simulink model "TypeA_siso180515"  (R2017b)
settings: Solver=ode45  StartTime=0.0  StopTime=12.0  RelTol=1e-3  EnableMultiTasking=on
undefined symbols (not defined in the file): cMat_BF, cMat_IM, cMat_MN, cMat_TM, gain_actBFGAS, gain_actBFL, gain_actBFP, gain_actBFR, gain_actBFT, gain_actBFV, gain_actBFY, gain_actF0GAS, gain_actF1GAS, gain_actF2GAS, gain_actF3GAS, gain_actIML, gain_actIMP, gain_actIMR, gain_actIMT, gain_actIMV, gain_actIMY, gain_actIPL, gain_actIPT, gain_actIPY, gain_actMNL, gain_actMNP, gain_actMNR, gain_actMNT, gain_actMNV, gain_actMNY, gain_actTML, gain_actTMP, gain_actTMY, gainBFGAS, gainBFL, gainBFP, gainBFR, gainBFT, gainBFV, gainBFY, gainF0GAS, gainF1GAS, gainF2GAS, gainF3GAS, gainHieBFP, gainHieBFR, gainHieBFY, gainHieIML, gainHieIMP, gainHieIMY, gainHieIPL, gainHieIPY, gainHieMNL, gainHieMNP, gainHieMNY, gainIML, gainIMP, gainIMR, gainIMT, gainIMV ... (+24)
libraries: cstblocks x57
(part 2 of 2)

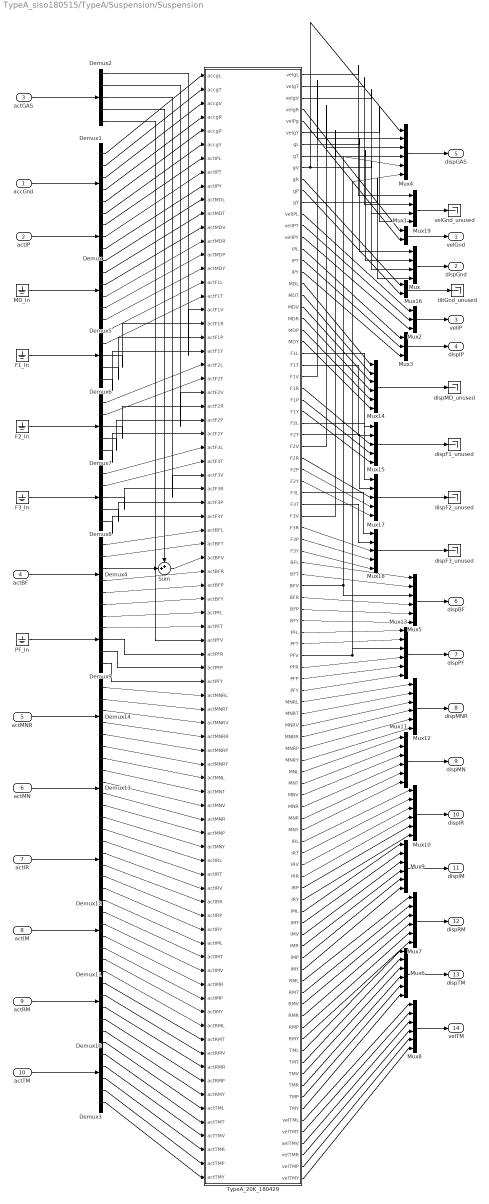
== system TypeA_siso180515/TypeA/Suspension/Suspension ==
  accGnd : Inport
  actIP : Inport  Port=2
  actGAS : Inport  Port=3
  actBF : Inport  Port=4
  actMNR : Inport  Port=5
  actMN : Inport  Port=6
  actIR : Inport  Port=7
  actIM : Inport  Port=8
  actRM : Inport  Port=9
  actTM : Inport  Port=10
  Demux : Demux  Outputs=3
  Demux{1,3..5,10..14} (9 alike) : Demux  Outputs=6
  Demux{2,6..9} (5 alike) : Demux  Outputs=5
  F1_In : Ground
  F2_In : Ground
  F3_In : Ground
  MD_In : Ground
  Mux : Mux
  Mux1 : Mux  Inputs=2
  Mux{4..14} (11 alike) : Mux  Inputs=6
  Mux15 : Mux  Inputs=5
  Mux16 : Mux  Inputs=2
  Mux17 : Mux  Inputs=5
  Mux18 : Mux  Inputs=5
  Mux19 : Mux
  Mux2 : Mux  Inputs=3
  Mux3 : Mux  Inputs=3
  PF_In : Ground
  Sum : Sum  Inputs=++|
  TypeA_20K_180429 : Subsystem
  dispF1_unused : Terminator
  dispF2_unused : Terminator
  dispF3_unused : Terminator
  dispMD_unused : Terminator
  tiltGnd_unused : Terminator
  velGnd_unused : Terminator
  velGnd : Outport
  dispGnd : Outport  Port=2
  velIP : Outport  Port=3
  dispIP : Outport  Port=4
  dispGAS : Outport  Port=5
  dispBF : Outport  Port=6
  dispPF : Outport  Port=7
  dispMNR : Outport  Port=8
  dispMN : Outport  Port=9
  dispIR : Outport  Port=10
  dispIM : Outport  Port=11
  dispRM : Outport  Port=12
  dispTM : Outport  Port=13
  velTM : Outport  Port=14
  wires:
  Mux/1 -> dispGnd/1
  Mux1/1 -> velGnd/1
  Mux2/1 -> velIP/1
  Mux3/1 -> dispIP/1
  Mux4/1 -> dispGAS/1
  Mux5/1 -> dispBF/1
  Mux6/1 -> dispTM/1
  actIP/1 -> Demux/1
  accGnd/1 -> Demux1/1
  actTM/1 -> Demux3/1
  Demux4/3 -> Sum/2
  Demux2/4 -> Sum/1
  Demux2/5 -> TypeA_20K_180429/42(actPFV)
  actBF/1 -> Demux4/1
  actGAS/1 -> Demux2/1
  Demux1/3 -> TypeA_20K_180429/3(accgV)
  Demux1/1 -> TypeA_20K_180429/1(accgL)
  Demux1/2 -> TypeA_20K_180429/2(accgT)
  Demux1/4 -> TypeA_20K_180429/4(accgR)
  Demux1/5 -> TypeA_20K_180429/5(accgP)
  Demux1/6 -> TypeA_20K_180429/6(accgY)
  Demux/1 -> TypeA_20K_180429/7(actIPL)
  Demux/2 -> TypeA_20K_180429/8(actIPT)
  Demux/3 -> TypeA_20K_180429/9(actIPY)
  MD_In/1 -> Demux5/1
  Demux5/1 -> TypeA_20K_180429/10(actMDL)
  Demux5/2 -> TypeA_20K_180429/11(actMDT)
  Demux5/3 -> TypeA_20K_180429/12(actMDV)
  Demux5/4 -> TypeA_20K_180429/13(actMDR)
  Demux5/5 -> TypeA_20K_180429/14(actMDP)
  Demux5/6 -> TypeA_20K_180429/15(actMDY)
  Demux2/1 -> TypeA_20K_180429/18(actF1V)
  Demux2/2 -> TypeA_20K_180429/24(actF2V)
  Demux2/3 -> TypeA_20K_180429/30(actF3V)
  Sum/1 -> TypeA_20K_180429/36(actBFV)
  F1_In/1 -> Demux6/1
  Demux6/2 -> TypeA_20K_180429/17(actF1T)
  Demux6/1 -> TypeA_20K_180429/16(actF1L)
  Demux6/5 -> TypeA_20K_180429/21(actF1Y)
  Demux6/3 -> TypeA_20K_180429/19(actF1R)
  Demux6/4 -> TypeA_20K_180429/20(actF1P)
  F2_In/1 -> Demux7/1
  Demux7/1 -> TypeA_20K_180429/22(actF2L)
  Demux7/2 -> TypeA_20K_180429/23(actF2T)
  Demux7/3 -> TypeA_20K_180429/25(actF2R)
  Demux7/4 -> TypeA_20K_180429/26(actF2P)
  Demux7/5 -> TypeA_20K_180429/27(actF2Y)
  F3_In/1 -> Demux8/1
  Demux8/2 -> TypeA_20K_180429/29(actF3T)
  Demux8/1 -> TypeA_20K_180429/28(actF3L)
  Demux8/5 -> TypeA_20K_180429/33(actF3Y)
  Demux8/4 -> TypeA_20K_180429/32(actF3P)
  Demux8/3 -> TypeA_20K_180429/31(actF3R)
  Demux4/1 -> TypeA_20K_180429/34(actBFL)
  Demux4/2 -> TypeA_20K_180429/35(actBFT)
  Demux4/4 -> TypeA_20K_180429/37(actBFR)
  Demux4/5 -> TypeA_20K_180429/38(actBFP)
  Demux4/6 -> TypeA_20K_180429/39(actBFY)
  PF_In/1 -> Demux9/1
  Demux9/1 -> TypeA_20K_180429/40(actPFL)
  Demux9/2 -> TypeA_20K_180429/41(actPFT)
  Demux9/4 -> TypeA_20K_180429/44(actPFP)
  Demux9/3 -> TypeA_20K_180429/43(actPFR)
  Demux9/5 -> TypeA_20K_180429/45(actPFY)
  actRM/1 -> Demux10/1
  actIM/1 -> Demux11/1
  actIR/1 -> Demux12/1
  actMN/1 -> Demux13/1
  actMNR/1 -> Demux14/1
  Demux14/4 -> TypeA_20K_180429/49(actMNRR)
  Demux14/5 -> TypeA_20K_180429/50(actMNRP)
  Demux14/6 -> TypeA_20K_180429/51(actMNRY)
  Demux14/1 -> TypeA_20K_180429/46(actMNRL)
  Demux14/2 -> TypeA_20K_180429/47(actMNRT)
  Demux14/3 -> TypeA_20K_180429/48(actMNRV)
  Demux13/2 -> TypeA_20K_180429/53(actMNT)
  Demux13/1 -> TypeA_20K_180429/52(actMNL)
  Demux13/3 -> TypeA_20K_180429/54(actMNV)
  Demux13/5 -> TypeA_20K_180429/56(actMNP)
  Demux13/4 -> TypeA_20K_180429/55(actMNR)
  Demux13/6 -> TypeA_20K_180429/57(actMNY)
  Demux12/6 -> TypeA_20K_180429/63(actIRY)
  Demux12/2 -> TypeA_20K_180429/59(actIRT)
  Demux12/5 -> TypeA_20K_180429/62(actIRP)
  Demux12/3 -> TypeA_20K_180429/60(actIRV)
  Demux12/4 -> TypeA_20K_180429/61(actIRR)
  Demux12/1 -> TypeA_20K_180429/58(actIRL)
  Demux11/2 -> TypeA_20K_180429/65(actIMT)
  Demux11/3 -> TypeA_20K_180429/66(actIMV)
  Demux11/5 -> TypeA_20K_180429/68(actIMP)
  Demux11/4 -> TypeA_20K_180429/67(actIMR)
  Demux11/1 -> TypeA_20K_180429/64(actIML)
  Demux11/6 -> TypeA_20K_180429/69(actIMY)
  Demux10/5 -> TypeA_20K_180429/74(actRMP)
  Demux10/6 -> TypeA_20K_180429/75(actRMY)
  Demux10/4 -> TypeA_20K_180429/73(actRMR)
  Demux10/3 -> TypeA_20K_180429/72(actRMV)
  Demux10/1 -> TypeA_20K_180429/70(actRML)
  Demux10/2 -> TypeA_20K_180429/71(actRMT)
  Demux3/3 -> TypeA_20K_180429/78(actTMV)
  Demux3/1 -> TypeA_20K_180429/76(actTML)
  Demux3/2 -> TypeA_20K_180429/77(actTMT)
  Demux3/4 -> TypeA_20K_180429/79(actTMR)
  Demux3/5 -> TypeA_20K_180429/80(actTMP)
  Demux3/6 -> TypeA_20K_180429/81(actTMY)
  Mux7/1 -> dispRM/1
  Mux8/1 -> velTM/1
  Mux9/1 -> dispIM/1
  Mux10/1 -> dispIR/1
  Mux11/1 -> dispMN/1
  Mux12/1 -> dispMNR/1
  Mux13/1 -> dispPF/1
  Mux14/1 -> dispMD_unused/1
  Mux15/1 -> dispF1_unused/1
  Mux16/1 -> tiltGnd_unused/1
  Mux17/1 -> dispF2_unused/1
  Mux18/1 -> dispF3_unused/1
  TypeA_20K_180429/4(velgR) -> Mux1/1
  TypeA_20K_180429/5(velPg) -> Mux1/2
  TypeA_20K_180429/8(gT) -> Mux/2
  TypeA_20K_180429/7(gL) -> Mux/1
  TypeA_20K_180429/9(gV) -> Mux/3, Mux4/1
  TypeA_20K_180429/11(gP) -> Mux16/2
  TypeA_20K_180429/10(gR) -> Mux16/1
  TypeA_20K_180429/12(gY) -> Mux/4
  TypeA_20K_180429/14(velIPT) -> Mux2/2
  TypeA_20K_180429/15(velIPY) -> Mux2/3
  TypeA_20K_180429/13(velIPL) -> Mux2/1
  TypeA_20K_180429/17(IPT) -> Mux3/2
  TypeA_20K_180429/16(IPL) -> Mux3/1
  TypeA_20K_180429/18(IPY) -> Mux3/3
  TypeA_20K_180429/19(MDL) -> Mux14/1
  TypeA_20K_180429/21(MDV) -> Mux14/3
  TypeA_20K_180429/20(MDT) -> Mux14/2
  TypeA_20K_180429/22(MDR) -> Mux14/4
  TypeA_20K_180429/23(MDP) -> Mux14/5
  TypeA_20K_180429/24(MDY) -> Mux14/6
  TypeA_20K_180429/27(F1V) -> Mux4/2
  TypeA_20K_180429/33(F2V) -> Mux4/3
  TypeA_20K_180429/39(F3V) -> Mux4/4
  TypeA_20K_180429/45(BFV) -> Mux4/5, Mux5/3
  TypeA_20K_180429/51(PFV) -> Mux4/6, Mux13/3
  TypeA_20K_180429/25(F1L) -> Mux15/1
  TypeA_20K_180429/26(F1T) -> Mux15/2
  TypeA_20K_180429/30(F1Y) -> Mux15/5
  TypeA_20K_180429/28(F1R) -> Mux15/3
  TypeA_20K_180429/29(F1P) -> Mux15/4
  TypeA_20K_180429/31(F2L) -> Mux17/1
  TypeA_20K_180429/32(F2T) -> Mux17/2
  TypeA_20K_180429/34(F2R) -> Mux17/3
  TypeA_20K_180429/36(F2Y) -> Mux17/5
  TypeA_20K_180429/35(F2P) -> Mux17/4
  TypeA_20K_180429/37(F3L) -> Mux18/1
  TypeA_20K_180429/38(F3T) -> Mux18/2
  TypeA_20K_180429/42(F3Y) -> Mux18/5
  TypeA_20K_180429/41(F3P) -> Mux18/4
  TypeA_20K_180429/40(F3R) -> Mux18/3
  TypeA_20K_180429/47(BFP) -> Mux5/5
  TypeA_20K_180429/48(BFY) -> Mux5/6
  TypeA_20K_180429/46(BFR) -> Mux5/4
  TypeA_20K_180429/44(BFT) -> Mux5/2
  TypeA_20K_180429/43(BFL) -> Mux5/1
  TypeA_20K_180429/54(PFY) -> Mux13/6
  TypeA_20K_180429/49(PFL) -> Mux13/1
  TypeA_20K_180429/50(PFT) -> Mux13/2
  TypeA_20K_180429/52(PFR) -> Mux13/4
  TypeA_20K_180429/53(PFP) -> Mux13/5
  TypeA_20K_180429/56(MNRT) -> Mux12/2
  TypeA_20K_180429/60(MNRY) -> Mux12/6
  TypeA_20K_180429/57(MNRV) -> Mux12/3
  TypeA_20K_180429/58(MNRR) -> Mux12/4
  TypeA_20K_180429/55(MNRL) -> Mux12/1
  TypeA_20K_180429/59(MNRP) -> Mux12/5
  TypeA_20K_180429/64(MNR) -> Mux11/4
  TypeA_20K_180429/61(MNL) -> Mux11/1
  TypeA_20K_180429/63(MNV) -> Mux11/3
  TypeA_20K_180429/62(MNT) -> Mux11/2
  TypeA_20K_180429/66(MNY) -> Mux11/6
  TypeA_20K_180429/65(MNP) -> Mux11/5
  TypeA_20K_180429/71(IRP) -> Mux10/5
  TypeA_20K_180429/69(IRV) -> Mux10/3
  TypeA_20K_180429/72(IRY) -> Mux10/6
  TypeA_20K_180429/70(IRR) -> Mux10/4
  TypeA_20K_180429/68(IRT) -> Mux10/2
  TypeA_20K_180429/67(IRL) -> Mux10/1
  TypeA_20K_180429/73(IML) -> Mux9/1
  TypeA_20K_180429/75(IMV) -> Mux9/3
  TypeA_20K_180429/74(IMT) -> Mux9/2
  TypeA_20K_180429/76(IMR) -> Mux9/4
  TypeA_20K_180429/77(IMP) -> Mux9/5
  TypeA_20K_180429/78(IMY) -> Mux9/6
  TypeA_20K_180429/83(RMP) -> Mux7/5
  TypeA_20K_180429/84(RMY) -> Mux7/6
  TypeA_20K_180429/79(RML) -> Mux7/1
  TypeA_20K_180429/81(RMV) -> Mux7/3
  TypeA_20K_180429/80(RMT) -> Mux7/2
  TypeA_20K_180429/82(RMR) -> Mux7/4
  TypeA_20K_180429/85(TML) -> Mux6/1
  TypeA_20K_180429/86(TMT) -> Mux6/2
  TypeA_20K_180429/88(TMR) -> Mux6/4
  TypeA_20K_180429/87(TMV) -> Mux6/3
  TypeA_20K_180429/89(TMP) -> Mux6/5
  TypeA_20K_180429/90(TMY) -> Mux6/6
  TypeA_20K_180429/93(velTMV) -> Mux8/3
  TypeA_20K_180429/94(velTMR) -> Mux8/4
  TypeA_20K_180429/96(velTMY) -> Mux8/6
  TypeA_20K_180429/91(velTML) -> Mux8/1
  TypeA_20K_180429/95(velTMP) -> Mux8/5
  TypeA_20K_180429/92(velTMT) -> Mux8/2
  Mux19/1 -> velGnd_unused/1
  TypeA_20K_180429/1(velgL) -> Mux19/1
  TypeA_20K_180429/2(velgT) -> Mux19/2
  TypeA_20K_180429/3(velgV) -> Mux19/3
  TypeA_20K_180429/6(velgY) -> Mux19/4

== system TypeA_siso180515/TypeA/Suspension/aMatrix_BF ==
  aMat_in : Inport
  cMat_BF : Constant  Value=cMat_BF  VectorParams1D=off
  coupling_BF : Product  Multiplication=Matrix(*)
  actBF : Outport
  wires:
  coupling_BF/1 -> actBF/1
  aMat_in/1 -> coupling_BF/2
  cMat_BF/1 -> coupling_BF/1

== system TypeA_siso180515/TypeA/Suspension/aMatrix_GAS ==
  aMat_in : Inport
  Add{1..4} (4 alike) : Sum  Inputs=+-
  Demux4 : Demux  Outputs=5
  Mux3 : Mux  Inputs=5
  actGAS : Outport
  wires:
  aMat_in/1 -> Demux4/1
  Mux3/1 -> actGAS/1
  Add1/1 -> Mux3/1
  Add2/1 -> Mux3/2
  Demux4/3 -> Add3/1, Add2/2
  Demux4/2 -> Add1/2, Add2/1
  Demux4/1 -> Add1/1
  Demux4/5 -> Mux3/5, Add4/2
  Add4/1 -> Mux3/4
  Add3/1 -> Mux3/3
  Demux4/4 -> Add3/2, Add4/1

== system TypeA_siso180515/TypeA/Suspension/aMatrix_IM ==
  aMat_in : Inport
  Gain : Gain  Gain=-1
  cMat_IM : Constant  Value=cMat_IM  VectorParams1D=off
  coupling_IM : Product  Multiplication=Matrix(*)
  actIR : Outport
  actIM : Outport  Port=2
  wires:
  coupling_IM/1 -> actIM/1, Gain/1
  aMat_in/1 -> coupling_IM/2
  cMat_IM/1 -> coupling_IM/1
  Gain/1 -> actIR/1

== system TypeA_siso180515/TypeA/Suspension/aMatrix_MN ==
  aMat_in : Inport
  Gain : Gain  Gain=-1
  cMat_MN : Constant  Value=cMat_MN  VectorParams1D=off
  coupling_MN : Product  Multiplication=Matrix(*)
  actMNR : Outport
  actMN : Outport  Port=2
  wires:
  coupling_MN/1 -> actMN/1, Gain/1
  aMat_in/1 -> coupling_MN/2
  cMat_MN/1 -> coupling_MN/1
  Gain/1 -> actMNR/1

== system TypeA_siso180515/TypeA/Suspension/aMatrix_TM ==
  aMat_in : Inport
  Demux : Demux  Outputs=3
  Demux1 : Demux  Outputs=3
  Gain : Gain  Gain=-1
  Ground{,1..5} (6 alike) : Ground
  Mux : Mux  Inputs=6
  Mux1 : Mux  Inputs=6
  cMat_TM : Constant  Value=cMat_TM  VectorParams1D=off
  coupling_TM : Product  Multiplication=Matrix(*)
  actRM : Outport
  actTM : Outport  Port=2
  wires:
  coupling_TM/1 -> Demux1/1, Gain/1
  aMat_in/1 -> coupling_TM/2  "3DoF"
  cMat_TM/1 -> coupling_TM/1
  Gain/1 -> Demux/1
  Demux/1 -> Mux/1
  Demux/2 -> Mux/5
  Demux/3 -> Mux/6
  Demux1/1 -> Mux1/1
  Demux1/3 -> Mux1/6
  Demux1/2 -> Mux1/5
  Ground/1 -> Mux/2
  Ground1/1 -> Mux/3
  Ground2/1 -> Mux/4
  Ground4/1 -> Mux1/3
  Ground3/1 -> Mux1/2
  Ground5/1 -> Mux1/4
  Mux/1 -> actRM/1  "6DoF"
  Mux1/1 -> actTM/1  "6DoF"

== system TypeA_siso180515/TypeA/Suspension/sMatrix_BF_LVDT ==
  dispGnd : Inport
  dispBF : Inport  Port=2
  Add2 : Sum  Inputs=-+
  Demux : Demux
  Ground : Ground
  Ground1 : Ground
  Mux : Mux  Inputs=6
  BF_LVDT : Outport
  wires:
  Add2/1 -> BF_LVDT/1  "6DoF"
  dispBF/1 -> Add2/2  "6DoF"
  dispGnd/1 -> Demux/1  "4DoF"
  Demux/1 -> Mux/1  "L"
  Demux/2 -> Mux/2  "T"
  Demux/3 -> Mux/3  "V"
  Demux/4 -> Mux/6  "Y"
  Ground/1 -> Mux/4  "R"
  Ground1/1 -> Mux/5  "P"
  Mux/1 -> Add2/1

== system TypeA_siso180515/TypeA/Suspension/sMatrix_GAS_LVDT ==
  dispGAS : Inport
  Add{1..5} (5 alike) : Sum  Inputs=-+
  Demux4 : Demux  Outputs=6
  Mux3 : Mux  Inputs=5
  GAS_LVDT : Outport
  wires:
  dispGAS/1 -> Demux4/1
  Demux4/1 -> Add2/1  "VGnd = IPV"
  Demux4/2 -> Add1/1, Add2/2  "VF1"
  Demux4/3 -> Add1/2, Add3/1  "VF2"
  Demux4/4 -> Add4/1, Add3/2  "VF3"
  Add2/1 -> Mux3/1  "GASF0"
  Add1/1 -> Mux3/2  "GASF1"
  Add3/1 -> Mux3/3  "GASF2"
  Mux3/1 -> GAS_LVDT/1
  Demux4/5 -> Add5/1, Add4/2  "VBF"
  Demux4/6 -> Add5/2  "VPF"
  Add4/1 -> Mux3/4  "GASF3"
  Add5/1 -> Mux3/5  "GASBF"

== system TypeA_siso180515/TypeA/Suspension/sMatrix_IM_PS ==
  dispIR : Inport
  dispIM : Inport  Port=2
  Add2 : Sum  Inputs=-+
  IM_PS : Outport
  wires:
  Add2/1 -> IM_PS/1
  dispIM/1 -> Add2/2
  dispIR/1 -> Add2/1

== system TypeA_siso180515/TypeA/Suspension/sMatrix_IP_LVDT ==
  dispGnd : Inport
  dispIP : Inport  Port=2
  Add2 : Sum  Inputs=-+
  Demux : Demux
  Mux : Mux  Inputs=3
  Terminator : Terminator
  IP_LVDT : Outport
  wires:
  Add2/1 -> IP_LVDT/1
  dispIP/1 -> Add2/2
  dispGnd/1 -> Demux/1
  Demux/1 -> Mux/1  "L"
  Demux/2 -> Mux/2  "T"
  Demux/4 -> Mux/3  "Y"
  Demux/3 -> Terminator/1  "V"
  Mux/1 -> Add2/1

== system TypeA_siso180515/TypeA/Suspension/sMatrix_MN_OpLev ==
  dispMN : Inport
  Demux4 : Demux  Outputs=6
  Mux3 : Mux  Inputs=3
  dispMNL : Terminator
  dispMNT : Terminator
  dispMNV : Terminator
  MN_OpLev : Outport
  wires:
  dispMN/1 -> Demux4/1
  Mux3/1 -> MN_OpLev/1
  Demux4/1 -> dispMNL/1
  Demux4/2 -> dispMNT/1
  Demux4/3 -> dispMNV/1
  Demux4/4 -> Mux3/1
  Demux4/5 -> Mux3/2
  Demux4/6 -> Mux3/3

== system TypeA_siso180515/TypeA/Suspension/sMatrix_MN_PS ==
  dispMNR : Inport
  dispMN : Inport  Port=2
  Add2 : Sum  Inputs=-+
  MN_PS : Outport
  wires:
  Add2/1 -> MN_PS/1
  dispMN/1 -> Add2/2
  dispMNR/1 -> Add2/1

== system TypeA_siso180515/TypeA/Suspension/sMatrix_PF_OpLev ==
  dispPF : Inport
  Demux4 : Demux  Outputs=6
  Mux3 : Mux  Inputs=3
  dispLPF : Terminator
  dispTPF : Terminator
  dispVPF : Terminator
  OpLev_PF : Outport
  wires:
  dispPF/1 -> Demux4/1
  Mux3/1 -> OpLev_PF/1
  Demux4/1 -> dispLPF/1
  Demux4/2 -> dispTPF/1
  Demux4/3 -> dispVPF/1
  Demux4/4 -> Mux3/1
  Demux4/5 -> Mux3/2
  Demux4/6 -> Mux3/3

== system TypeA_siso180515/TypeA/Suspension/sMatrix_TM_OpLev ==
  dispTM : Inport
  Demux4 : Demux  Outputs=6
  Mux3 : Mux  Inputs=3
  dispTMR : Terminator
  dispTMT : Terminator
  dispTMV : Terminator
  TM_OpLev : Outport
  wires:
  dispTM/1 -> Demux4/1
  Mux3/1 -> TM_OpLev/1
  Demux4/1 -> Mux3/1
  Demux4/2 -> dispTMT/1
  Demux4/3 -> dispTMV/1
  Demux4/4 -> dispTMR/1
  Demux4/5 -> Mux3/2
  Demux4/6 -> Mux3/3

== system TypeA_siso180515/TypeA/Suspension/sMatrix_TM_PS ==
  dispRM : Inport
  dispTM : Inport  Port=2
  Add2 : Sum  Inputs=-+
  Demux : Demux  Outputs=6
  Demux1 : Demux  Outputs=6
  Mux : Mux  Inputs=3
  Mux1 : Mux  Inputs=3
  Terminator{,1..5} (6 alike) : Terminator
  TM_PS : Outport
  wires:
  Add2/1 -> TM_PS/1  "(L, P, Y)"
  dispRM/1 -> Demux/1
  dispTM/1 -> Demux1/1
  Demux/1 -> Mux/1  "L"
  Demux/5 -> Mux/2  "P"
  Demux/6 -> Mux/3  "Y"
  Demux1/1 -> Mux1/1  "L"
  Demux1/5 -> Mux1/2  "P"
  Demux1/6 -> Mux1/3  "Y"
  Mux/1 -> Add2/1
  Mux1/1 -> Add2/2
  Demux/2 -> Terminator/1  "T"
  Demux/4 -> Terminator2/1  "R"
  Demux/3 -> Terminator1/1  "V"
  Demux1/4 -> Terminator5/1  "R"
  Demux1/2 -> Terminator3/1  "T"
  Demux1/3 -> Terminator4/1  "V"

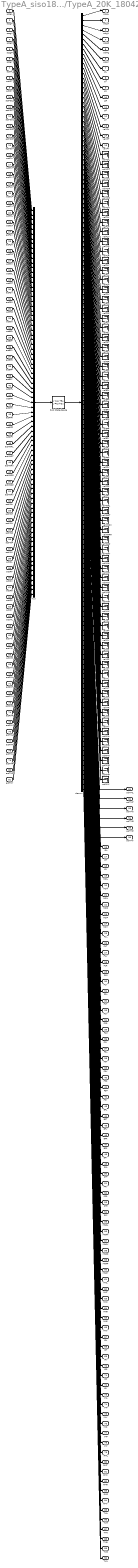
== system TypeA_siso180515/TypeA/Suspension/Suspension/TypeA_20K_180429 ==
  accgL : Inport
  accgT : Inport  Port=2
  accgV : Inport  Port=3
  accgR : Inport  Port=4
  accgP : Inport  Port=5
  accgY : Inport  Port=6
  actIPL : Inport  Port=7
  actIPT : Inport  Port=8
  actIPY : Inport  Port=9
  actMDL : Inport  Port=10
  actMDT : Inport  Port=11
  actMDV : Inport  Port=12
  actMDR : Inport  Port=13
  actMDP : Inport  Port=14
  actMDY : Inport  Port=15
  actF1L : Inport  Port=16
  actF1T : Inport  Port=17
  actF1V : Inport  Port=18
  actF1R : Inport  Port=19
  actF1P : Inport  Port=20
  actF1Y : Inport  Port=21
  actF2L : Inport  Port=22
  actF2T : Inport  Port=23
  actF2V : Inport  Port=24
  actF2R : Inport  Port=25
  actF2P : Inport  Port=26
  actF2Y : Inport  Port=27
  actF3L : Inport  Port=28
  actF3T : Inport  Port=29
  actF3V : Inport  Port=30
  actF3R : Inport  Port=31
  actF3P : Inport  Port=32
  actF3Y : Inport  Port=33
  actBFL : Inport  Port=34
  actBFT : Inport  Port=35
  actBFV : Inport  Port=36
  actBFR : Inport  Port=37
  actBFP : Inport  Port=38
  actBFY : Inport  Port=39
  actPFL : Inport  Port=40
  actPFT : Inport  Port=41
  actPFV : Inport  Port=42
  actPFR : Inport  Port=43
  actPFP : Inport  Port=44
  actPFY : Inport  Port=45
  actMNRL : Inport  Port=46
  actMNRT : Inport  Port=47
  actMNRV : Inport  Port=48
  actMNRR : Inport  Port=49
  actMNRP : Inport  Port=50
  actMNRY : Inport  Port=51
  actMNL : Inport  Port=52
  actMNT : Inport  Port=53
  actMNV : Inport  Port=54
  actMNR : Inport  Port=55
  actMNP : Inport  Port=56
  actMNY : Inport  Port=57
  actIRL : Inport  Port=58
  actIRT : Inport  Port=59
  actIRV : Inport  Port=60
  actIRR : Inport  Port=61
  actIRP : Inport  Port=62
  actIRY : Inport  Port=63
  actIML : Inport  Port=64
  actIMT : Inport  Port=65
  actIMV : Inport  Port=66
  actIMR : Inport  Port=67
  actIMP : Inport  Port=68
  actIMY : Inport  Port=69
  actRML : Inport  Port=70
  actRMT : Inport  Port=71
  actRMV : Inport  Port=72
  actRMR : Inport  Port=73
  actRMP : Inport  Port=74
  actRMY : Inport  Port=75
  actTML : Inport  Port=76
  actTMT : Inport  Port=77
  actTMV : Inport  Port=78
  actTMR : Inport  Port=79
  actTMP : Inport  Port=80
  actTMY : Inport  Port=81
  SAS State-Space : StateSpace  A=sys1.A  B=sys1.B  C=sys1.C  D=sys1.D  InitialCondition=0  ContinuousStateAttributes='SUS_SS_MODEL'
  demux : Demux  Outputs=162
  mux : Mux  Inputs=81
  velBFL : Terminator
  velBFP : Terminator
  velBFR : Terminator
  velBFT : Terminator
  velBFV : Terminator
  velBFY : Terminator
  velF1L : Terminator
  velF1P : Terminator
  velF1R : Terminator
  velF1T : Terminator
  velF1V : Terminator
  velF1Y : Terminator
  velF2L : Terminator
  velF2P : Terminator
  velF2R : Terminator
  velF2T : Terminator
  velF2V : Terminator
  velF2Y : Terminator
  velF3L : Terminator
  velF3P : Terminator
  velF3R : Terminator
  velF3T : Terminator
  velF3V : Terminator
  velF3Y : Terminator
  velIML : Terminator
  velIMP : Terminator
  velIMR : Terminator
  velIMT : Terminator
  velIMV : Terminator
  velIMY : Terminator
  velIRL : Terminator
  velIRP : Terminator
  velIRR : Terminator
  velIRT : Terminator
  velIRV : Terminator
  velIRY : Terminator
  velMDL : Terminator
  velMDP : Terminator
  velMDR : Terminator
  velMDT : Terminator
  velMDV : Terminator
  velMDY : Terminator
  velMNL : Terminator
  velMNP : Terminator
  velMNR : Terminator
  velMNRL : Terminator
  velMNRP : Terminator
  velMNRR : Terminator
  velMNRT : Terminator
  velMNRV : Terminator
  velMNRY : Terminator
  velMNT : Terminator
  velMNV : Terminator
  velMNY : Terminator
  velPFL : Terminator
  velPFP : Terminator
  velPFR : Terminator
  velPFT : Terminator
  velPFV : Terminator
  velPFY : Terminator
  velRML : Terminator
  velRMP : Terminator
  velRMR : Terminator
  velRMT : Terminator
  velRMV : Terminator
  velRMY : Terminator
  velgL : Outport
  velgT : Outport  Port=2
  velgV : Outport  Port=3
  velgR : Outport  Port=4
  velPg : Outport  Port=5
  velgY : Outport  Port=6
  gL : Outport  Port=7
  gT : Outport  Port=8
  gV : Outport  Port=9
  gR : Outport  Port=10
  gP : Outport  Port=11
  gY : Outport  Port=12
  velIPL : Outport  Port=13
  velIPT : Outport  Port=14
  velIPY : Outport  Port=15
  IPL : Outport  Port=16
  IPT : Outport  Port=17
  IPY : Outport  Port=18
  MDL : Outport  Port=19
  MDT : Outport  Port=20
  MDV : Outport  Port=21
  MDR : Outport  Port=22
  MDP : Outport  Port=23
  MDY : Outport  Port=24
  F1L : Outport  Port=25
  F1T : Outport  Port=26
  F1V : Outport  Port=27
  F1R : Outport  Port=28
  F1P : Outport  Port=29
  F1Y : Outport  Port=30
  F2L : Outport  Port=31
  F2T : Outport  Port=32
  F2V : Outport  Port=33
  F2R : Outport  Port=34
  F2P : Outport  Port=35
  F2Y : Outport  Port=36
  F3L : Outport  Port=37
  F3T : Outport  Port=38
  F3V : Outport  Port=39
  F3R : Outport  Port=40
  F3P : Outport  Port=41
  F3Y : Outport  Port=42
  BFL : Outport  Port=43
  BFT : Outport  Port=44
  BFV : Outport  Port=45
  BFR : Outport  Port=46
  BFP : Outport  Port=47
  BFY : Outport  Port=48
  PFL : Outport  Port=49
  PFT : Outport  Port=50
  PFV : Outport  Port=51
  PFR : Outport  Port=52
  PFP : Outport  Port=53
  PFY : Outport  Port=54
  MNRL : Outport  Port=55
  MNRT : Outport  Port=56
  MNRV : Outport  Port=57
  MNRR : Outport  Port=58
  MNRP : Outport  Port=59
  MNRY : Outport  Port=60
  MNL : Outport  Port=61
  MNT : Outport  Port=62
  MNV : Outport  Port=63
  MNR : Outport  Port=64
  MNP : Outport  Port=65
  MNY : Outport  Port=66
  IRL : Outport  Port=67
  IRT : Outport  Port=68
  IRV : Outport  Port=69
  IRR : Outport  Port=70
  IRP : Outport  Port=71
  IRY : Outport  Port=72
  IML : Outport  Port=73
  IMT : Outport  Port=74
  IMV : Outport  Port=75
  IMR : Outport  Port=76
  IMP : Outport  Port=77
  IMY : Outport  Port=78
  RML : Outport  Port=79
  RMT : Outport  Port=80
  RMV : Outport  Port=81
  RMR : Outport  Port=82
  RMP : Outport  Port=83
  RMY : Outport  Port=84
  TML : Outport  Port=85
  TMT : Outport  Port=86
  TMV : Outport  Port=87
  TMR : Outport  Port=88
  TMP : Outport  Port=89
  TMY : Outport  Port=90
  velTML : Outport  Port=91
  velTMT : Outport  Port=92
  velTMV : Outport  Port=93
  velTMR : Outport  Port=94
  velTMP : Outport  Port=95
  velTMY : Outport  Port=96
  wires:
  mux/1 -> SAS State-Space/1
  SAS State-Space/1 -> demux/1
  accgL/1 -> mux/1
  accgT/1 -> mux/2
  accgV/1 -> mux/3
  accgR/1 -> mux/4
  accgP/1 -> mux/5
  accgY/1 -> mux/6
  actIPL/1 -> mux/7
  actIPT/1 -> mux/8
  actIPY/1 -> mux/9
  actMDL/1 -> mux/10
  actMDT/1 -> mux/11
  actMDV/1 -> mux/12
  actMDR/1 -> mux/13
  actMDP/1 -> mux/14
  actMDY/1 -> mux/15
  actF1L/1 -> mux/16
  actF1T/1 -> mux/17
  actF1V/1 -> mux/18
  actF1R/1 -> mux/19
  actF1P/1 -> mux/20
  actF1Y/1 -> mux/21
  actF2L/1 -> mux/22
  actF2T/1 -> mux/23
  actF2V/1 -> mux/24
  actF2R/1 -> mux/25
  actF2P/1 -> mux/26
  actF2Y/1 -> mux/27
  actF3L/1 -> mux/28
  actF3T/1 -> mux/29
  actF3V/1 -> mux/30
  actF3R/1 -> mux/31
  actF3P/1 -> mux/32
  actF3Y/1 -> mux/33
  actBFL/1 -> mux/34
  actBFT/1 -> mux/35
  actBFV/1 -> mux/36
  actBFR/1 -> mux/37
  actBFP/1 -> mux/38
  actBFY/1 -> mux/39
  actPFL/1 -> mux/40
  actPFT/1 -> mux/41
  actPFV/1 -> mux/42
  actPFR/1 -> mux/43
  actPFP/1 -> mux/44
  actPFY/1 -> mux/45
  actMNRL/1 -> mux/46
  actMNRT/1 -> mux/47
  actMNRV/1 -> mux/48
  actMNRR/1 -> mux/49
  actMNRP/1 -> mux/50
  actMNRY/1 -> mux/51
  actMNL/1 -> mux/52
  actMNT/1 -> mux/53
  actMNV/1 -> mux/54
  actMNR/1 -> mux/55
  actMNP/1 -> mux/56
  actMNY/1 -> mux/57
  actIRL/1 -> mux/58
  actIRT/1 -> mux/59
  actIRV/1 -> mux/60
  actIRR/1 -> mux/61
  actIRP/1 -> mux/62
  actIRY/1 -> mux/63
  actIML/1 -> mux/64
  actIMT/1 -> mux/65
  actIMV/1 -> mux/66
  actIMR/1 -> mux/67
  actIMP/1 -> mux/68
  actIMY/1 -> mux/69
  actRML/1 -> mux/70
  actRMT/1 -> mux/71
  actRMV/1 -> mux/72
  actRMR/1 -> mux/73
  actRMP/1 -> mux/74
  actRMY/1 -> mux/75
  actTML/1 -> mux/76
  actTMT/1 -> mux/77
  actTMV/1 -> mux/78
  actTMR/1 -> mux/79
  actTMP/1 -> mux/80
  actTMY/1 -> mux/81
  demux/1 -> velgL/1
  demux/2 -> velgT/1
  demux/3 -> velgV/1
  demux/4 -> velgR/1
  demux/5 -> velPg/1
  demux/6 -> velgY/1
  demux/7 -> gL/1
  demux/8 -> gT/1
  demux/9 -> gV/1
  demux/10 -> gR/1
  demux/11 -> gP/1
  demux/12 -> gY/1
  demux/13 -> velIPL/1
  demux/14 -> velIPT/1
  demux/15 -> velIPY/1
  demux/16 -> velMDL/1
  demux/17 -> velMDT/1
  demux/18 -> velMDV/1
  demux/19 -> velMDR/1
  demux/20 -> velMDP/1
  demux/21 -> velMDY/1
  demux/22 -> velF1L/1
  demux/23 -> velF1T/1
  demux/24 -> velF1V/1
  demux/25 -> velF1R/1
  demux/26 -> velF1P/1
  demux/27 -> velF1Y/1
  demux/28 -> velF2L/1
  demux/29 -> velF2T/1
  demux/30 -> velF2V/1
  demux/31 -> velF2R/1
  demux/32 -> velF2P/1
  demux/33 -> velF2Y/1
  demux/34 -> velF3L/1
  demux/35 -> velF3T/1
  demux/36 -> velF3V/1
  demux/37 -> velF3R/1
  demux/38 -> velF3P/1
  demux/39 -> velF3Y/1
  demux/40 -> velBFL/1
  demux/41 -> velBFT/1
  demux/42 -> velBFV/1
  demux/43 -> velBFR/1
  demux/44 -> velBFP/1
  demux/45 -> velBFY/1
  demux/46 -> velPFL/1
  demux/47 -> velPFT/1
  demux/48 -> velPFV/1
  demux/49 -> velPFR/1
  demux/50 -> velPFP/1
  demux/51 -> velPFY/1
  demux/52 -> velMNRL/1
  demux/53 -> velMNRT/1
  demux/54 -> velMNRV/1
  demux/55 -> velMNRR/1
  demux/56 -> velMNRP/1
  demux/57 -> velMNRY/1
  demux/58 -> velMNL/1
  demux/59 -> velMNT/1
  demux/60 -> velMNV/1
  demux/61 -> velMNR/1
  demux/62 -> velMNP/1
  demux/63 -> velMNY/1
  demux/64 -> velIRL/1
  demux/65 -> velIRT/1
  demux/66 -> velIRV/1
  demux/67 -> velIRR/1
  demux/68 -> velIRP/1
  demux/69 -> velIRY/1
  demux/70 -> velIML/1
  demux/71 -> velIMT/1
  demux/72 -> velIMV/1
  demux/73 -> velIMR/1
  demux/74 -> velIMP/1
  demux/75 -> velIMY/1
  demux/76 -> velRML/1
  demux/77 -> velRMT/1
  demux/78 -> velRMV/1
  demux/79 -> velRMR/1
  demux/80 -> velRMP/1
  demux/81 -> velRMY/1
  demux/82 -> velTML/1
  demux/83 -> velTMT/1
  demux/84 -> velTMV/1
  demux/85 -> velTMR/1
  demux/86 -> velTMP/1
  demux/87 -> velTMY/1
  demux/88 -> IPL/1
  demux/89 -> IPT/1
  demux/90 -> IPY/1
  demux/91 -> MDL/1
  demux/92 -> MDT/1
  demux/93 -> MDV/1
  demux/94 -> MDR/1
  demux/95 -> MDP/1
  demux/96 -> MDY/1
  demux/97 -> F1L/1
  demux/98 -> F1T/1
  demux/99 -> F1V/1
  demux/100 -> F1R/1
  demux/101 -> F1P/1
  demux/102 -> F1Y/1
  demux/103 -> F2L/1
  demux/104 -> F2T/1
  demux/105 -> F2V/1
  demux/106 -> F2R/1
  demux/107 -> F2P/1
  demux/108 -> F2Y/1
  demux/109 -> F3L/1
  demux/110 -> F3T/1
  demux/111 -> F3V/1
  demux/112 -> F3R/1
  demux/113 -> F3P/1
  demux/114 -> F3Y/1
  demux/115 -> BFL/1
  demux/116 -> BFT/1
  demux/117 -> BFV/1
  demux/118 -> BFR/1
  demux/119 -> BFP/1
  demux/120 -> BFY/1
  demux/121 -> PFL/1
  demux/122 -> PFT/1
  demux/123 -> PFV/1
  demux/124 -> PFR/1
  demux/125 -> PFP/1
  demux/126 -> PFY/1
  demux/127 -> MNRL/1
  demux/128 -> MNRT/1
  demux/129 -> MNRV/1
  demux/130 -> MNRR/1
  demux/131 -> MNRP/1
  demux/132 -> MNRY/1
  demux/133 -> MNL/1
  demux/134 -> MNT/1
  demux/135 -> MNV/1
  demux/136 -> MNR/1
  demux/137 -> MNP/1
  demux/138 -> MNY/1
  demux/139 -> IRL/1
  demux/140 -> IRT/1
  demux/141 -> IRV/1
  demux/142 -> IRR/1
  demux/143 -> IRP/1
  demux/144 -> IRY/1
  demux/145 -> IML/1
  demux/146 -> IMT/1
  demux/147 -> IMV/1
  demux/148 -> IMR/1
  demux/149 -> IMP/1
  demux/150 -> IMY/1
  demux/151 -> RML/1
  demux/152 -> RMT/1
  demux/153 -> RMV/1
  demux/154 -> RMR/1
  demux/155 -> RMP/1
  demux/156 -> RMY/1
  demux/157 -> TML/1
  demux/158 -> TMT/1
  demux/159 -> TMV/1
  demux/160 -> TMR/1
  demux/161 -> TMP/1
  demux/162 -> TMY/1
